simulink model "simsamolot"  (R2021b)
settings: Solver=VariableStepAuto  StartTime=0.0  StopTime=50  RelTol=1e-3
undefined symbols (not defined in the file or in its folder): DiscIntNeverNeededParam
libraries: simulink x1, fuzblock x1
settings Model: Creator=mateu  LastModifiedBy=mateu

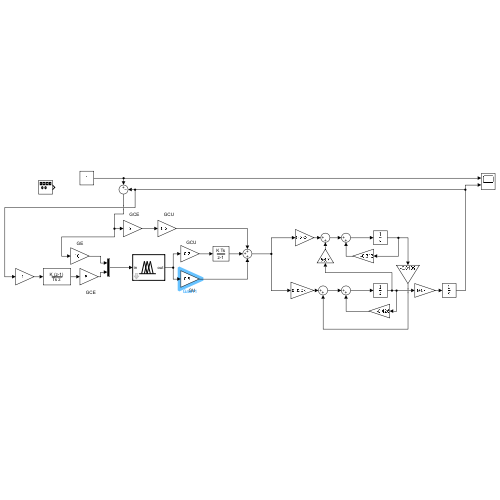
[thumbnail: Simulink's stored preview of the top-level diagram]
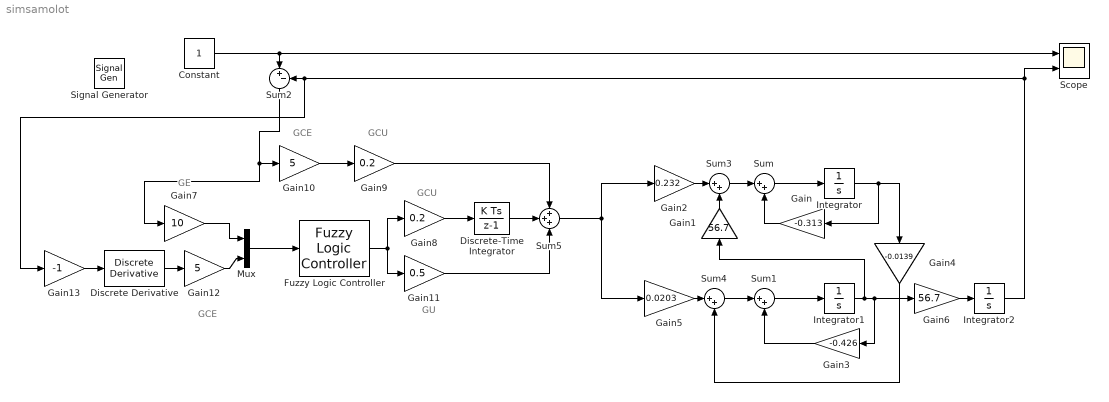
== system simsamolot ==
  note: GCE
  note: GE
  note: GCE
  note: GCU
  note: GU
  note: GCU
  Constant : Constant
  Discrete Derivative : simulink/Discrete/Discrete Derivative  gainval=1.0  ICPrevScaledInput=0.0  OutMin=[]  OutMax=[]  OutDataType=fixdt(1, 16)  OutScaling=2^-10  DoSatur=off
  Discrete-Time Integrator : DiscreteIntegrator  SampleTime=-1  ICPrevOutput=DiscIntNeverNeededParam  ICPrevScaledInput=DiscIntNeverNeededParam
  Fuzzy Logic Controller : fuzblock/Fuzzy Logic  Controller  FIS=fsamolot  OutputSampleNumber=101  DataType=double  FuzzifiedInputs=off  RuleFiringStrengths=off  RuleOutputs=off  AggregatedOutputs=off  SimulateUsing=Interpreted execution  OutOfRangeInputValueMessage=warning  NoRuleFiredMessage=warning  EmptyOutputFuzzySetMessage=warning
  Gain : Gain  Gain=-0.313
  Gain1 : Gain  Gain=56.7
  Gain10 : Gain  Gain=5
  Gain11 : Gain  Gain=0.5
  Gain12 : Gain  Gain=5
  Gain13 : Gain  Gain=-1
  Gain2 : Gain  Gain=0.232
  Gain3 : Gain  Gain=-0.426
  Gain4 : Gain  Gain=-0.0139
  Gain5 : Gain  Gain=0.0203
  Gain6 : Gain  Gain=56.7
  Gain7 : Gain  Gain=10
  Gain8 : Gain  Gain=0.2
  Gain9 : Gain  Gain=0.2
  Integrator : Integrator
  Integrator1 : Integrator
  Integrator2 : Integrator
  Mux : Mux  Inputs=2
  Scope : Scope  NumInputPorts=2
  Signal Generator : SignalGenerator  WaveForm=square
  Sum{,1,3..4} (4 alike) : Sum  Inputs=|++
  Sum2 : Sum  Inputs=|+-
  Sum5 : Sum  Inputs=+++
  wires:
  Sum/1 -> Integrator/1
  Sum1/1 -> Integrator1/1
  Gain/1 -> Sum/2
  Integrator/1 -> Gain4/1, Gain/1
  Sum3/1 -> Sum/1
  Gain1/1 -> Sum3/2
  Gain2/1 -> Sum3/1
  Integrator1/1 -> Gain6/1, Gain3/1, Gain1/1
  Gain3/1 -> Sum1/2
  Sum4/1 -> Sum1/1
  Gain4/1 -> Sum4/2
  Gain5/1 -> Sum4/1
  Gain6/1 -> Integrator2/1
  Integrator2/1 -> Scope/2, Gain13/1, Sum2/2
  Constant/1 -> Scope/1, Sum2/1
  Gain10/1 -> Gain9/1
  Gain13/1 -> Discrete Derivative/1
  Discrete Derivative/1 -> Gain12/1
  Gain12/1 -> Mux/2
  Gain7/1 -> Mux/1
  Fuzzy Logic Controller/1 -> Gain11/1, Gain8/1
  Gain8/1 -> Discrete-Time Integrator/1
  Discrete-Time Integrator/1 -> Sum5/2
  Sum5/1 -> Gain5/1, Gain2/1
  Gain11/1 -> Sum5/3
  Gain9/1 -> Sum5/1
  Mux/1 -> Fuzzy Logic Controller/1
  Sum2/1 -> Gain7/1, Gain10/1
